simulink model "smx_controlesPID1"  (R2017b)
settings: Solver=VariableStepAuto  StartTime=0.0  StopTime=20  RelTol=1e-2
undefined symbols (not defined in the file): ts
libraries: cstblocks x2
settings Model: Creator=Martin  LastModifiedBy=Martin

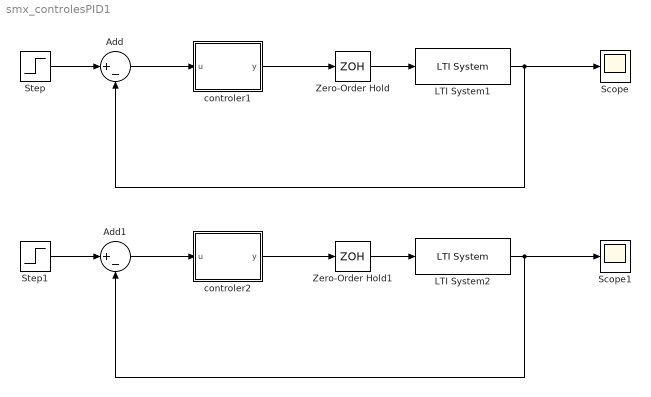
== system smx_controlesPID1 ==
  Add : Sum  Inputs=|+-
  Add1 : Sum  Inputs=|+-
  LTI System1 : cstblocks/LTI System  sys=tf1  IC=[]
  LTI System2 : cstblocks/LTI System  sys=tf1  IC=[]
  Scope : Scope
  Scope1 : Scope
  Step : Step  SampleTime=0
  Step1 : Step  SampleTime=0
  Zero-Order Hold : ZeroOrderHold  SampleTime=ts
  Zero-Order Hold1 : ZeroOrderHold  SampleTime=ts*2
  controler1 : Subsystem
  controler2 : Subsystem
  wires:
  Step/1 -> Add/1
  Zero-Order Hold/1 -> LTI System1/1
  LTI System1/1 -> Scope/1, Add/2
  controler1/1(y) -> Zero-Order Hold/1
  Add/1 -> controler1/1(u)
  Add1/1 -> controler2/1(u)
  LTI System2/1 -> Add1/2, Scope1/1
  Zero-Order Hold1/1 -> LTI System2/1
  Step1/1 -> Add1/1
  controler2/1(y) -> Zero-Order Hold1/1

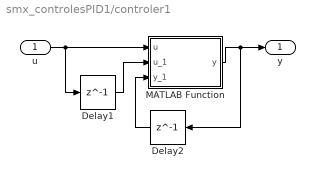
== system smx_controlesPID1/controler1 ==
  u : Inport
  Delay1 : Delay  DelayLength=1
  Delay2 : Delay  DelayLength=1
  MATLAB Function : MATLAB Function  TreatAsAtomicUnit=on
  y : Outport
  wires:
  Delay2/1 -> MATLAB Function/3(y_1)
  Delay1/1 -> MATLAB Function/2(u_1)
  MATLAB Function/1(y) -> y/1, Delay2/1
  u/1 -> MATLAB Function/1(u), Delay1/1

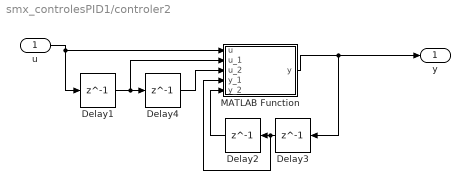
== system smx_controlesPID1/controler2 ==
  u : Inport
  Delay{1..4} (4 alike) : Delay  DelayLength=1
  MATLAB Function : MATLAB Function  TreatAsAtomicUnit=on
  y : Outport
  wires:
  u/1 -> Delay1/1, MATLAB Function/1(u)
  MATLAB Function/1(y) -> Delay3/1, y/1
  Delay1/1 -> MATLAB Function/2(u_1), Delay4/1
  Delay3/1 -> MATLAB Function/4(y_1), Delay2/1
  Delay4/1 -> MATLAB Function/3(u_2)
  Delay2/1 -> MATLAB Function/5(y_2)

== matlab function smx_controlesPID1/controler2/MATLAB Function ==
  data: u input; y output; u_1 input; u_2 input; y_1 input; y_2 input
function y = fcn(u, u_1, u_2, y_1, y_2)

y = -1.474*u + 1.473*u_1 - 0*u_2 + 1*y_1 - 0*y_2;

== matlab function smx_controlesPID1/controler1/MATLAB Function ==
  data: u input; y output; u_1 input; y_1 input
function y = fcn(u, u_1, y_1)

y = -1.471*u + 1.47*u_1 + y_1;
